simulink model "test"  (R2021b)
settings: Solver=VariableStepAuto  StartTime=0.0  StopTime=10  RelTol=1e-3
settings Model: Creator=philippsum  LastModifiedBy=philippsum

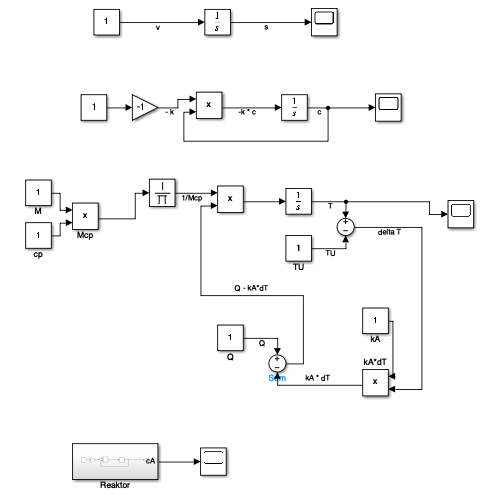
[thumbnail: Simulink's stored preview of the top-level diagram]
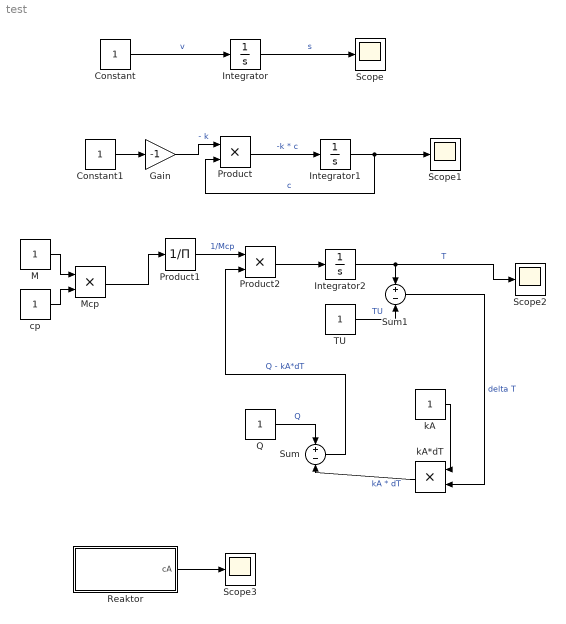
== system test ==
  Constant : Constant
  Constant1 : Constant
  Gain : Gain  Gain=-1
  Integrator : Integrator
  Integrator1 : Integrator  InitialCondition=10
  Integrator2 : Integrator
  M : Constant
  Mcp : Product
  Product : Product
  Product1 : Product  Inputs=/
  Product2 : Product
  Q : Constant
  Reaktor : Subsystem
  Scope{,1..3} (4 alike) : Scope
  Sum : Sum  Inputs=+-
  Sum1 : Sum  Inputs=+-
  TU : Constant
  cp : Constant
  kA : Constant
  kA*dT : Product
  wires:
  Constant/1 -> Integrator/1  "v"
  Integrator/1 -> Scope/1  "s"
  Constant1/1 -> Gain/1
  Gain/1 -> Product/1  "- k"
  Product/1 -> Integrator1/1  "-k * c"
  Integrator1/1 -> Scope1/1, Product/2  "c"
  Product1/1 -> Product2/1  "1/Mcp"
  Q/1 -> Sum/1  "Q"
  M/1 -> Mcp/1
  cp/1 -> Mcp/2
  Mcp/1 -> Product1/1
  Sum/1 -> Product2/2  "Q - kA*dT"
  Product2/1 -> Integrator2/1
  Integrator2/1 -> Scope2/1, Sum1/1  "T"
  TU/1 -> Sum1/2  "TU"
  kA/1 -> kA*dT/1
  Sum1/1 -> kA*dT/2  "delta T"
  kA*dT/1 -> Sum/2  "kA * dT"
  Reaktor/1(cA) -> Scope3/1

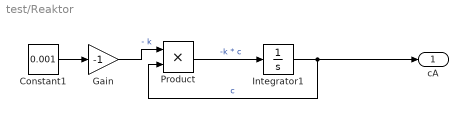
== system test/Reaktor ==
  Constant1 : Constant  Value=0.001
  Gain : Gain  Gain=-1
  Integrator1 : Integrator  InitialCondition=1.5
  Product : Product
  cA : Outport
  wires:
  Constant1/1 -> Gain/1
  Product/1 -> Integrator1/1  "-k * c"
  Integrator1/1 -> cA/1, Product/2  "c"
  Gain/1 -> Product/1  "- k"
